simulink library "inp"  (R2021b)
settings: Solver=VariableStepAuto  StartTime=0.0  StopTime=10.0  RelTol=1e-3
undefined symbols (not defined in the file): C_TASK_5MS_S, FALSE, KINP_AcoreReadyToSlp_flg_ovrdflg, KINP_AcoreReadyToSlp_flg_ovrdval, KINP_AllowMovThd_OTA_enum_ovrdflg, KINP_AllowMovThd_OTA_enum_ovrdval, KINP_APSAngleTarget_Deg_ovrdflg, KINP_APSAngleTarget_Deg_ovrdval, KINP_APSDecReq_mps2_ovrdflg, KINP_APSDecReq_mps2_ovrdval, KINP_APSDecReqA_flg_ovrdflg, KINP_APSDecReqA_flg_ovrdval, KINP_APSDFLL_cm_ovrdflg, KINP_APSDFLL_cm_ovrdval, KINP_APSDFLR_cm_ovrdflg, KINP_APSDFLR_cm_ovrdval, KINP_APSDRLL_cm_ovrdflg, KINP_APSDRLL_cm_ovrdval, KINP_APSDRLR_cm_ovrdflg, KINP_APSDRLR_cm_ovrdval, KINP_APSExitCondition_enum_ovrdflg, KINP_APSExitCondition_enum_ovrdval, KINP_APSHWVer_enum_ovrdflg, KINP_APSHWVer_enum_ovrdval, KINP_APSProgressPCT_pct_ovrdflg, KINP_APSProgressPCT_pct_ovrdval, KINP_APSPwrReq_enum_ovrdflg, KINP_APSPwrReq_enum_ovrdval, KINP_APSReq_enum_ovrdflg, KINP_APSReq_enum_ovrdval, KINP_APSRQDisplay_enum_ovrdflg, KINP_APSRQDisplay_enum_ovrdval, KINP_APSRqEPASCtrl_flg_ovrdflg, KINP_APSRqEPASCtrl_flg_ovrdval, KINP_APSShiftPosnReq_enum_ovrdval, KINP_APSShiftPosnReq_enum_ovrflg, KINP_APSSpeedCMD_kph_ovrdval, KINP_APSSpeedCMD_kph_ovrflg, KINP_APSStaSystem_enum_ovrdflg, KINP_APSStaSystem_enum_ovrdval, KINP_APSSWVer_enum_ovrdflg, KINP_APSSWVer_enum_ovrdval, KINP_APSVMCReqA_flg_ovrdval, KINP_APSVMCReqA_flg_ovrflg, KINP_APSVRqEPASCtrl_flg_ovrdflg, KINP_APSVRqEPASCtrl_flg_ovrdval, KINP_AuxBattVolmV_mV_ovrdflg, KINP_AuxBattVolmV_mV_ovrdval, KINP_CAASSta_enum_ovrdflg, KINP_CAASSta_enum_ovrdval, KINP_CAASVMCReqA_flg_ovrdval, KINP_CAASVMCReqA_flg_ovrflg, KINP_CAN1BusOff_flg_ovrdflg, KINP_CAN1BusOff_flg_ovrdval, KINP_CAN2BusOff_flg_ovrdflg, KINP_CAN2BusOff_flg_ovrdval, KINP_CAN3BusOff_flg_ovrdflg, KINP_CAN3BusOff_flg_ovrdval, KINP_CAN4BusOff_flg_ovrdflg, KINP_CAN4BusOff_flg_ovrdval ... (+152)
libraries: FVT_lib x1037, hcu_lib x1
(part 25 of 34)

== system inp/INP/CAN3/SignalCheck/Shifter2 ==
  BHAL_outputs : Inport
  inp_CanValid_bus : Inport  Port=2
  CSW2DimSwSta : FVT_lib/inp/can_signal_template  SystemSampleTime=-1  VariantActivationTime=update diagram  Latency=0  AutoFrameSizeCalculation=off
      link override defval: Value=KINP_CSW2DimSwSta_flg_defval
      link override ovrdflg: Value=KINP_CSW2DimSwSta_flg_ovrdflg
      link override ovrdval: Value=KINP_CSW2DimSwSta_flg_ovrdval
  CSW2FWasSwSta : FVT_lib/inp/can_signal_template  SystemSampleTime=-1  VariantActivationTime=update diagram  Latency=0  AutoFrameSizeCalculation=off
      link override defval: Value=KINP_CSW2FWasSwSta_enum_defval
      link override ovrdflg: Value=KINP_CSW2FWasSwSta_enum_ovrdflg
      link override ovrdval: Value=KINP_CSW2FWasSwSta_enum_ovrdval
  CSW2FWipSwSta : FVT_lib/inp/can_signal_template  SystemSampleTime=-1  VariantActivationTime=update diagram  Latency=0  AutoFrameSizeCalculation=off
      link override defval: Value=KINP_CSW2FWipSwSta_enum_defval
      link override ovrdflg: Value=KINP_CSW2FWipSwSta_enum_ovrdflg
      link override ovrdval: Value=KINP_CSW2FWipSwSta_enum_ovrdval
  CSW2PassSWSta : FVT_lib/inp/can_signal_template  SystemSampleTime=-1  VariantActivationTime=update diagram  Latency=0  AutoFrameSizeCalculation=off
      link override defval: Value=KINP_CSW2PassSWSta_flg_defval
      link override ovrdflg: Value=KINP_CSW2PassSWSta_flg_ovrdflg
      link override ovrdval: Value=KINP_CSW2PassSWSta_flg_ovrdval
  CSW2RWipWasSwSta : FVT_lib/inp/can_signal_template  SystemSampleTime=-1  VariantActivationTime=update diagram  Latency=0  AutoFrameSizeCalculation=off
      link override defval: Value=KINP_CSW2RWipWasSwSta_enum_defval
      link override ovrdflg: Value=KINP_CSW2RWipWasSwSta_enum_ovrdflg
      link override ovrdval: Value=KINP_CSW2RWipWasSwSta_enum_ovrdval
  CSW2TurnSwSta : FVT_lib/inp/can_signal_template  SystemSampleTime=-1  VariantActivationTime=update diagram  Latency=0  AutoFrameSizeCalculation=off
      link override defval: Value=KINP_CSW2TurnSwSta_enum_defval
      link override ovrdflg: Value=KINP_CSW2TurnSwSta_enum_ovrdflg
      link override ovrdval: Value=KINP_CSW2TurnSwSta_enum_ovrdval
  Shifter2CSErr : FVT_lib/inp/can_signal_template  SystemSampleTime=-1  VariantActivationTime=update diagram  Latency=0  AutoFrameSizeCalculation=off
      link override defval: Value=KINP_Shifter2CSErr_flg_defval
      link override ovrdflg: Value=KINP_Shifter2CSErr_flg_ovrdflg
      link override ovrdval: Value=KINP_Shifter2CSErr_flg_ovrdval
  Shifter2RCErr : FVT_lib/inp/can_signal_template  SystemSampleTime=-1  VariantActivationTime=update diagram  Latency=0  AutoFrameSizeCalculation=off
      link override defval: Value=KINP_Shifter2RCErr_flg_defval
      link override ovrdflg: Value=KINP_Shifter2RCErr_flg_ovrdflg
      link override ovrdval: Value=KINP_Shifter2RCErr_flg_ovrdval
  Terminator_{1..8} (8 alike) : Terminator
  True_VHAL_CSW2DimSwSta_flg : Constant  Value=TRUE  OutDataTypeStr=boolean
  True_VHAL_CSW2FWasSwSta_enum : Constant  Value=TRUE  OutDataTypeStr=boolean
  True_VHAL_CSW2FWipSwSta_enum : Constant  Value=TRUE  OutDataTypeStr=boolean
  True_VHAL_CSW2PassSWSta_flg : Constant  Value=TRUE  OutDataTypeStr=boolean
  True_VHAL_CSW2RWipWasSwSta_enum : Constant  Value=TRUE  OutDataTypeStr=boolean
  True_VHAL_CSW2TurnSwSta_enum : Constant  Value=TRUE  OutDataTypeStr=boolean
  True_VHAL_Shifter2CSErr_flg : Constant  Value=TRUE  OutDataTypeStr=boolean
  True_VHAL_Shifter2RCErr_flg : Constant  Value=TRUE  OutDataTypeStr=boolean
  slr1_{1..8} (8 alike) : BusSelector  OutputSignals=VINP_CANMsgValidShifter2_flg
  slr_VHAL_CSW2DimSwSta_flg : BusSelector  OutputSignals=VHAL_CSW2DimSwSta_flg
  slr_VHAL_CSW2FWasSwSta_enum : BusSelector  OutputSignals=VHAL_CSW2FWasSwSta_enum
  slr_VHAL_CSW2FWipSwSta_enum : BusSelector  OutputSignals=VHAL_CSW2FWipSwSta_enum
  slr_VHAL_CSW2PassSWSta_flg : BusSelector  OutputSignals=VHAL_CSW2PassSWSta_flg
  slr_VHAL_CSW2RWipWasSwSta_enum : BusSelector  OutputSignals=VHAL_CSW2RWipWasSwSta_enum
  slr_VHAL_CSW2TurnSwSta_enum : BusSelector  OutputSignals=VHAL_CSW2TurnSwSta_enum
  slr_VHAL_Shifter2CSErr_flg : BusSelector  OutputSignals=VHAL_Shifter2CSErr_flg
  slr_VHAL_Shifter2RCErr_flg : BusSelector  OutputSignals=VHAL_Shifter2RCErr_flg
  VINP_Shifter2CSErr_flg : Outport
  VINP_Shifter2RCErr_flg : Outport  Port=2
  VINP_CSW2DimSwSta_flg : Outport  Port=3
  VINP_CSW2FWasSwSta_enum : Outport  Port=4
  VINP_CSW2FWipSwSta_enum : Outport  Port=5
  VINP_CSW2PassSWSta_flg : Outport  Port=6
  VINP_CSW2RWipWasSwSta_enum : Outport  Port=7
  VINP_CSW2TurnSwSta_enum : Outport  Port=8
  wires:
  BHAL_outputs/1 -> [BHAL_outputs]
  inp_CanValid_bus/1 -> [inp_CanValid_bus]
  [BHAL_outputs] -> slr_VHAL_Shifter2CSErr_flg/1
  slr_VHAL_Shifter2CSErr_flg/1 -> Shifter2CSErr/1  "<VHAL_Shifter2CSErr_flg>"
  True_VHAL_Shifter2CSErr_flg/1 -> Shifter2CSErr/2
  [inp_CanValid_bus] -> slr1_1/1
  slr1_1/1 -> Shifter2CSErr/3  "<VINP_CANMsgValidShifter2_flg>"
  Shifter2CSErr/1 -> VINP_Shifter2CSErr_flg/1  "VINP_Shifter2CSErr_flg"
  Shifter2CSErr/2 -> Terminator_1/1
  [BHAL_outputs] -> slr_VHAL_Shifter2RCErr_flg/1
  slr_VHAL_Shifter2RCErr_flg/1 -> Shifter2RCErr/1  "<VHAL_Shifter2RCErr_flg>"
  True_VHAL_Shifter2RCErr_flg/1 -> Shifter2RCErr/2
  [inp_CanValid_bus] -> slr1_2/1
  slr1_2/1 -> Shifter2RCErr/3  "<VINP_CANMsgValidShifter2_flg>"
  Shifter2RCErr/1 -> VINP_Shifter2RCErr_flg/1  "VINP_Shifter2RCErr_flg"
  Shifter2RCErr/2 -> Terminator_2/1
  [BHAL_outputs] -> slr_VHAL_CSW2DimSwSta_flg/1
  slr_VHAL_CSW2DimSwSta_flg/1 -> CSW2DimSwSta/1  "<VHAL_CSW2DimSwSta_flg>"
  True_VHAL_CSW2DimSwSta_flg/1 -> CSW2DimSwSta/2
  [inp_CanValid_bus] -> slr1_3/1
  slr1_3/1 -> CSW2DimSwSta/3  "<VINP_CANMsgValidShifter2_flg>"
  CSW2DimSwSta/1 -> VINP_CSW2DimSwSta_flg/1  "VINP_CSW2DimSwSta_flg"
  CSW2DimSwSta/2 -> Terminator_3/1
  [BHAL_outputs] -> slr_VHAL_CSW2FWasSwSta_enum/1
  slr_VHAL_CSW2FWasSwSta_enum/1 -> CSW2FWasSwSta/1  "<VHAL_CSW2FWasSwSta_enum>"
  True_VHAL_CSW2FWasSwSta_enum/1 -> CSW2FWasSwSta/2
  [inp_CanValid_bus] -> slr1_4/1
  slr1_4/1 -> CSW2FWasSwSta/3  "<VINP_CANMsgValidShifter2_flg>"
  CSW2FWasSwSta/1 -> VINP_CSW2FWasSwSta_enum/1  "VINP_CSW2FWasSwSta_enum"
  CSW2FWasSwSta/2 -> Terminator_4/1
  [BHAL_outputs] -> slr_VHAL_CSW2FWipSwSta_enum/1
  slr_VHAL_CSW2FWipSwSta_enum/1 -> CSW2FWipSwSta/1  "<VHAL_CSW2FWipSwSta_enum>"
  True_VHAL_CSW2FWipSwSta_enum/1 -> CSW2FWipSwSta/2
  [inp_CanValid_bus] -> slr1_5/1
  slr1_5/1 -> CSW2FWipSwSta/3  "<VINP_CANMsgValidShifter2_flg>"
  CSW2FWipSwSta/1 -> VINP_CSW2FWipSwSta_enum/1  "VINP_CSW2FWipSwSta_enum"
  CSW2FWipSwSta/2 -> Terminator_5/1
  [BHAL_outputs] -> slr_VHAL_CSW2PassSWSta_flg/1
  slr_VHAL_CSW2PassSWSta_flg/1 -> CSW2PassSWSta/1  "<VHAL_CSW2PassSWSta_flg>"
  True_VHAL_CSW2PassSWSta_flg/1 -> CSW2PassSWSta/2
  [inp_CanValid_bus] -> slr1_6/1
  slr1_6/1 -> CSW2PassSWSta/3  "<VINP_CANMsgValidShifter2_flg>"
  CSW2PassSWSta/1 -> VINP_CSW2PassSWSta_flg/1  "VINP_CSW2PassSWSta_flg"
  CSW2PassSWSta/2 -> Terminator_6/1
  [BHAL_outputs] -> slr_VHAL_CSW2RWipWasSwSta_enum/1
  slr_VHAL_CSW2RWipWasSwSta_enum/1 -> CSW2RWipWasSwSta/1  "<VHAL_CSW2RWipWasSwSta_enum>"
  True_VHAL_CSW2RWipWasSwSta_enum/1 -> CSW2RWipWasSwSta/2
  [inp_CanValid_bus] -> slr1_7/1
  slr1_7/1 -> CSW2RWipWasSwSta/3  "<VINP_CANMsgValidShifter2_flg>"
  CSW2RWipWasSwSta/1 -> VINP_CSW2RWipWasSwSta_enum/1  "VINP_CSW2RWipWasSwSta_enum"
  CSW2RWipWasSwSta/2 -> Terminator_7/1
  [BHAL_outputs] -> slr_VHAL_CSW2TurnSwSta_enum/1
  slr_VHAL_CSW2TurnSwSta_enum/1 -> CSW2TurnSwSta/1  "<VHAL_CSW2TurnSwSta_enum>"
  True_VHAL_CSW2TurnSwSta_enum/1 -> CSW2TurnSwSta/2
  [inp_CanValid_bus] -> slr1_8/1
  slr1_8/1 -> CSW2TurnSwSta/3  "<VINP_CANMsgValidShifter2_flg>"
  CSW2TurnSwSta/1 -> VINP_CSW2TurnSwSta_enum/1  "VINP_CSW2TurnSwSta_enum"
  CSW2TurnSwSta/2 -> Terminator_8/1

== system inp/INP/CAN4/SignalCheck/BodyZone_DR1 ==
  BHAL_outputs : Inport
  inp_CanValid_bus : Inport  Port=2
  BDDSEATAntiSta : FVT_lib/inp/can_signal_template  SystemSampleTime=-1  VariantActivationTime=update diagram  Latency=0  AutoFrameSizeCalculation=off
      link override defval: Value=KINP_BDDSEATAntiSta_flg_defval
      link override ovrdflg: Value=KINP_BDDSEATAntiSta_flg_ovrdflg
      link override ovrdval: Value=KINP_BDDSEATAntiSta_flg_ovrdval
  BDDSEATEntryFunSta : FVT_lib/inp/can_signal_template  SystemSampleTime=-1  VariantActivationTime=update diagram  Latency=0  AutoFrameSizeCalculation=off
      link override defval: Value=KINP_BDDSEATEntryFunSta_flg_defval
      link override ovrdflg: Value=KINP_BDDSEATEntryFunSta_flg_ovrdflg
      link override ovrdval: Value=KINP_BDDSEATEntryFunSta_flg_ovrdval
  BDDSEATErrorSta : FVT_lib/inp/can_signal_template  SystemSampleTime=-1  VariantActivationTime=update diagram  Latency=0  AutoFrameSizeCalculation=off
      link override defval: Value=KINP_BDDSEATErrorSta_flg_defval
      link override ovrdflg: Value=KINP_BDDSEATErrorSta_flg_ovrdflg
      link override ovrdval: Value=KINP_BDDSEATErrorSta_flg_ovrdval
  BDDSEATMemSetSta : FVT_lib/inp/can_signal_template  SystemSampleTime=-1  VariantActivationTime=update diagram  Latency=0  AutoFrameSizeCalculation=off
      link override defval: Value=KINP_BDDSEATMemSetSta_enum_defval
      link override ovrdflg: Value=KINP_BDDSEATMemSetSta_enum_ovrdflg
      link override ovrdval: Value=KINP_BDDSEATMemSetSta_enum_ovrdval
  BDDSEATModeSta : FVT_lib/inp/can_signal_template  SystemSampleTime=-1  VariantActivationTime=update diagram  Latency=0  AutoFrameSizeCalculation=off
      link override defval: Value=KINP_BDDSEATModeSta_enum_defval
      link override ovrdflg: Value=KINP_BDDSEATModeSta_enum_ovrdflg
      link override ovrdval: Value=KINP_BDDSEATModeSta_enum_ovrdval
  BDDSEATVentSta : FVT_lib/inp/can_signal_template  SystemSampleTime=-1  VariantActivationTime=update diagram  Latency=0  AutoFrameSizeCalculation=off
      link override defval: Value=KINP_BDDSEATVentSta_enum_defval
      link override ovrdflg: Value=KINP_BDDSEATVentSta_enum_ovrdflg
      link override ovrdval: Value=KINP_BDDSEATVentSta_enum_ovrdval
  BDDSEATheaterSta : FVT_lib/inp/can_signal_template  SystemSampleTime=-1  VariantActivationTime=update diagram  Latency=0  AutoFrameSizeCalculation=off
      link override defval: Value=KINP_BDDSEATheaterSta_enum_defval
      link override ovrdflg: Value=KINP_BDDSEATheaterSta_enum_ovrdflg
      link override ovrdval: Value=KINP_BDDSEATheaterSta_enum_ovrdval
  Terminator_{1..7} (7 alike) : Terminator
  True_VHAL_BDDSEATAntiSta_flg : Constant  Value=TRUE  OutDataTypeStr=boolean
  True_VHAL_BDDSEATEntryFunSta_flg : Constant  Value=TRUE  OutDataTypeStr=boolean
  True_VHAL_BDDSEATErrorSta_flg : Constant  Value=TRUE  OutDataTypeStr=boolean
  True_VHAL_BDDSEATMemSetSta_enum : Constant  Value=TRUE  OutDataTypeStr=boolean
  True_VHAL_BDDSEATModeSta_enum : Constant  Value=TRUE  OutDataTypeStr=boolean
  True_VHAL_BDDSEATVentSta_enum : Constant  Value=TRUE  OutDataTypeStr=boolean
  True_VHAL_BDDSEATheaterSta_enum : Constant  Value=TRUE  OutDataTypeStr=boolean
  slr1_{1..7} (7 alike) : BusSelector  OutputSignals=VINP_CANMsgValidBodyZoneDR1_flg
  slr_VHAL_BDDSEATAntiSta_flg : BusSelector  OutputSignals=VHAL_BDDSEATAntiSta_flg
  slr_VHAL_BDDSEATEntryFunSta_flg : BusSelector  OutputSignals=VHAL_BDDSEATEntryFunSta_flg
  slr_VHAL_BDDSEATErrorSta_flg : BusSelector  OutputSignals=VHAL_BDDSEATErrorSta_flg
  slr_VHAL_BDDSEATMemSetSta_enum : BusSelector  OutputSignals=VHAL_BDDSEATMemSetSta_enum
  slr_VHAL_BDDSEATModeSta_enum : BusSelector  OutputSignals=VHAL_BDDSEATModeSta_enum
  slr_VHAL_BDDSEATVentSta_enum : BusSelector  OutputSignals=VHAL_BDDSEATVentSta_enum
  slr_VHAL_BDDSEATheaterSta_enum : BusSelector  OutputSignals=VHAL_BDDSEATheaterSta_enum
  VINP_BDDSEATAntiSta_flg : Outport
  VINP_BDDSEATEntryFunSta_flg : Outport  Port=2
  VINP_BDDSEATErrorSta_flg : Outport  Port=3
  VINP_BDDSEATMemSetSta_enum : Outport  Port=4
  VINP_BDDSEATModeSta_enum : Outport  Port=5
  VINP_BDDSEATVentSta_enum : Outport  Port=6
  VINP_BDDSEATheaterSta_enum : Outport  Port=7
  wires:
  BHAL_outputs/1 -> [BHAL_outputs]
  inp_CanValid_bus/1 -> [inp_CanValid_bus]
  [BHAL_outputs] -> slr_VHAL_BDDSEATAntiSta_flg/1
  slr_VHAL_BDDSEATAntiSta_flg/1 -> BDDSEATAntiSta/1  "<VHAL_BDDSEATAntiSta_flg>"
  True_VHAL_BDDSEATAntiSta_flg/1 -> BDDSEATAntiSta/2
  [inp_CanValid_bus] -> slr1_1/1
  slr1_1/1 -> BDDSEATAntiSta/3  "<VINP_CANMsgValidBodyZoneDR1_flg>"
  BDDSEATAntiSta/1 -> VINP_BDDSEATAntiSta_flg/1  "VINP_BDDSEATAntiSta_flg"
  BDDSEATAntiSta/2 -> Terminator_1/1
  [BHAL_outputs] -> slr_VHAL_BDDSEATEntryFunSta_flg/1
  slr_VHAL_BDDSEATEntryFunSta_flg/1 -> BDDSEATEntryFunSta/1  "<VHAL_BDDSEATEntryFunSta_flg>"
  True_VHAL_BDDSEATEntryFunSta_flg/1 -> BDDSEATEntryFunSta/2
  [inp_CanValid_bus] -> slr1_2/1
  slr1_2/1 -> BDDSEATEntryFunSta/3  "<VINP_CANMsgValidBodyZoneDR1_flg>"
  BDDSEATEntryFunSta/1 -> VINP_BDDSEATEntryFunSta_flg/1  "VINP_BDDSEATEntryFunSta_flg"
  BDDSEATEntryFunSta/2 -> Terminator_2/1
  [BHAL_outputs] -> slr_VHAL_BDDSEATErrorSta_flg/1
  slr_VHAL_BDDSEATErrorSta_flg/1 -> BDDSEATErrorSta/1  "<VHAL_BDDSEATErrorSta_flg>"
  True_VHAL_BDDSEATErrorSta_flg/1 -> BDDSEATErrorSta/2
  [inp_CanValid_bus] -> slr1_3/1
  slr1_3/1 -> BDDSEATErrorSta/3  "<VINP_CANMsgValidBodyZoneDR1_flg>"
  BDDSEATErrorSta/1 -> VINP_BDDSEATErrorSta_flg/1  "VINP_BDDSEATErrorSta_flg"
  BDDSEATErrorSta/2 -> Terminator_3/1
  [BHAL_outputs] -> slr_VHAL_BDDSEATMemSetSta_enum/1
  slr_VHAL_BDDSEATMemSetSta_enum/1 -> BDDSEATMemSetSta/1  "<VHAL_BDDSEATMemSetSta_enum>"
  True_VHAL_BDDSEATMemSetSta_enum/1 -> BDDSEATMemSetSta/2
  [inp_CanValid_bus] -> slr1_4/1
  slr1_4/1 -> BDDSEATMemSetSta/3  "<VINP_CANMsgValidBodyZoneDR1_flg>"
  BDDSEATMemSetSta/1 -> VINP_BDDSEATMemSetSta_enum/1  "VINP_BDDSEATMemSetSta_enum"
  BDDSEATMemSetSta/2 -> Terminator_4/1
  [BHAL_outputs] -> slr_VHAL_BDDSEATModeSta_enum/1
  slr_VHAL_BDDSEATModeSta_enum/1 -> BDDSEATModeSta/1  "<VHAL_BDDSEATModeSta_enum>"
  True_VHAL_BDDSEATModeSta_enum/1 -> BDDSEATModeSta/2
  [inp_CanValid_bus] -> slr1_5/1
  slr1_5/1 -> BDDSEATModeSta/3  "<VINP_CANMsgValidBodyZoneDR1_flg>"
  BDDSEATModeSta/1 -> VINP_BDDSEATModeSta_enum/1  "VINP_BDDSEATModeSta_enum"
  BDDSEATModeSta/2 -> Terminator_5/1
  [BHAL_outputs] -> slr_VHAL_BDDSEATVentSta_enum/1
  slr_VHAL_BDDSEATVentSta_enum/1 -> BDDSEATVentSta/1  "<VHAL_BDDSEATVentSta_enum>"
  True_VHAL_BDDSEATVentSta_enum/1 -> BDDSEATVentSta/2
  [inp_CanValid_bus] -> slr1_6/1
  slr1_6/1 -> BDDSEATVentSta/3  "<VINP_CANMsgValidBodyZoneDR1_flg>"
  BDDSEATVentSta/1 -> VINP_BDDSEATVentSta_enum/1  "VINP_BDDSEATVentSta_enum"
  BDDSEATVentSta/2 -> Terminator_6/1
  [BHAL_outputs] -> slr_VHAL_BDDSEATheaterSta_enum/1
  slr_VHAL_BDDSEATheaterSta_enum/1 -> BDDSEATheaterSta/1  "<VHAL_BDDSEATheaterSta_enum>"
  True_VHAL_BDDSEATheaterSta_enum/1 -> BDDSEATheaterSta/2
  [inp_CanValid_bus] -> slr1_7/1
  slr1_7/1 -> BDDSEATheaterSta/3  "<VINP_CANMsgValidBodyZoneDR1_flg>"
  BDDSEATheaterSta/1 -> VINP_BDDSEATheaterSta_enum/1  "VINP_BDDSEATheaterSta_enum"
  BDDSEATheaterSta/2 -> Terminator_7/1

== system inp/INP/CAN4/SignalCheck/BodyZone_DR2 ==
  BHAL_outputs : Inport
  inp_CanValid_bus : Inport  Port=2
  BDAPMWinFOpenedSta : FVT_lib/inp/can_signal_template  SystemSampleTime=-1  VariantActivationTime=update diagram  Latency=0  AutoFrameSizeCalculation=off
      link override defval: Value=KINP_BDAPMWinFOpenedSta_pct_defval
      link override ovrdflg: Value=KINP_BDAPMWinFOpenedSta_pct_ovrdflg
      link override ovrdval: Value=KINP_BDAPMWinFOpenedSta_pct_ovrdval
  BDAPMWinROpenedSta : FVT_lib/inp/can_signal_template  SystemSampleTime=-1  VariantActivationTime=update diagram  Latency=0  AutoFrameSizeCalculation=off
      link override defval: Value=KINP_BDAPMWinROpenedSta_pct_defval
      link override ovrdflg: Value=KINP_BDAPMWinROpenedSta_pct_ovrdflg
      link override ovrdval: Value=KINP_BDAPMWinROpenedSta_pct_ovrdval
  BDDoorFHandleCloseSta : FVT_lib/inp/can_signal_template  SystemSampleTime=-1  VariantActivationTime=update diagram  Latency=0  AutoFrameSizeCalculation=off
      link override defval: Value=KINP_BDDoorFHandleCloseSta_flg_defval
      link override ovrdflg: Value=KINP_BDDoorFHandleCloseSta_flg_ovrdflg
      link override ovrdval: Value=KINP_BDDoorFHandleCloseSta_flg_ovrdval
  BDDoorRHandleCloseSta : FVT_lib/inp/can_signal_template  SystemSampleTime=-1  VariantActivationTime=update diagram  Latency=0  AutoFrameSizeCalculation=off
      link override defval: Value=KINP_BDDoorRHandleCloseSta_flg_defval
      link override ovrdflg: Value=KINP_BDDoorRHandleCloseSta_flg_ovrdflg
      link override ovrdval: Value=KINP_BDDoorRHandleCloseSta_flg_ovrdval
  Terminator_{1..4} (4 alike) : Terminator
  True_VHAL_BDAPMWinFOpenedSta_pct : Constant  Value=TRUE  OutDataTypeStr=boolean
  True_VHAL_BDAPMWinROpenedSta_pct : Constant  Value=TRUE  OutDataTypeStr=boolean
  True_VHAL_BDDoorFHandleCloseSta_flg : Constant  Value=TRUE  OutDataTypeStr=boolean
  True_VHAL_BDDoorRHandleCloseSta_flg : Constant  Value=TRUE  OutDataTypeStr=boolean
  slr1_{1..4} (4 alike) : BusSelector  OutputSignals=VINP_CANMsgValidBodyZoneDR2_flg
  slr_VHAL_BDAPMWinFOpenedSta_pct : BusSelector  OutputSignals=VHAL_BDAPMWinFOpenedSta_pct
  slr_VHAL_BDAPMWinROpenedSta_pct : BusSelector  OutputSignals=VHAL_BDAPMWinROpenedSta_pct
  slr_VHAL_BDDoorFHandleCloseSta_flg : BusSelector  OutputSignals=VHAL_BDDoorFHandleCloseSta_flg
  slr_VHAL_BDDoorRHandleCloseSta_flg : BusSelector  OutputSignals=VHAL_BDDoorRHandleCloseSta_flg
  VINP_BDAPMWinFOpenedSta_pct : Outport
  VINP_BDAPMWinROpenedSta_pct : Outport  Port=2
  VINP_BDDoorFHandleCloseSta_flg : Outport  Port=3
  VINP_BDDoorRHandleCloseSta_flg : Outport  Port=4
  wires:
  BHAL_outputs/1 -> [BHAL_outputs]
  inp_CanValid_bus/1 -> [inp_CanValid_bus]
  [BHAL_outputs] -> slr_VHAL_BDAPMWinFOpenedSta_pct/1
  slr_VHAL_BDAPMWinFOpenedSta_pct/1 -> BDAPMWinFOpenedSta/1  "<VHAL_BDAPMWinFOpenedSta_pct>"
  True_VHAL_BDAPMWinFOpenedSta_pct/1 -> BDAPMWinFOpenedSta/2
  [inp_CanValid_bus] -> slr1_1/1
  slr1_1/1 -> BDAPMWinFOpenedSta/3  "<VINP_CANMsgValidBodyZoneDR2_flg>"
  BDAPMWinFOpenedSta/1 -> VINP_BDAPMWinFOpenedSta_pct/1  "VINP_BDAPMWinFOpenedSta_pct"
  BDAPMWinFOpenedSta/2 -> Terminator_1/1
  [BHAL_outputs] -> slr_VHAL_BDAPMWinROpenedSta_pct/1
  slr_VHAL_BDAPMWinROpenedSta_pct/1 -> BDAPMWinROpenedSta/1  "<VHAL_BDAPMWinROpenedSta_pct>"
  True_VHAL_BDAPMWinROpenedSta_pct/1 -> BDAPMWinROpenedSta/2
  [inp_CanValid_bus] -> slr1_2/1
  slr1_2/1 -> BDAPMWinROpenedSta/3  "<VINP_CANMsgValidBodyZoneDR2_flg>"
  BDAPMWinROpenedSta/1 -> VINP_BDAPMWinROpenedSta_pct/1  "VINP_BDAPMWinROpenedSta_pct"
  BDAPMWinROpenedSta/2 -> Terminator_2/1
  [BHAL_outputs] -> slr_VHAL_BDDoorFHandleCloseSta_flg/1
  slr_VHAL_BDDoorFHandleCloseSta_flg/1 -> BDDoorFHandleCloseSta/1  "<VHAL_BDDoorFHandleCloseSta_flg>"
  True_VHAL_BDDoorFHandleCloseSta_flg/1 -> BDDoorFHandleCloseSta/2
  [inp_CanValid_bus] -> slr1_3/1
  slr1_3/1 -> BDDoorFHandleCloseSta/3  "<VINP_CANMsgValidBodyZoneDR2_flg>"
  BDDoorFHandleCloseSta/1 -> VINP_BDDoorFHandleCloseSta_flg/1  "VINP_BDDoorFHandleCloseSta_flg"
  BDDoorFHandleCloseSta/2 -> Terminator_3/1
  [BHAL_outputs] -> slr_VHAL_BDDoorRHandleCloseSta_flg/1
  slr_VHAL_BDDoorRHandleCloseSta_flg/1 -> BDDoorRHandleCloseSta/1  "<VHAL_BDDoorRHandleCloseSta_flg>"
  True_VHAL_BDDoorRHandleCloseSta_flg/1 -> BDDoorRHandleCloseSta/2
  [inp_CanValid_bus] -> slr1_4/1
  slr1_4/1 -> BDDoorRHandleCloseSta/3  "<VINP_CANMsgValidBodyZoneDR2_flg>"
  BDDoorRHandleCloseSta/1 -> VINP_BDDoorRHandleCloseSta_flg/1  "VINP_BDDoorRHandleCloseSta_flg"
  BDDoorRHandleCloseSta/2 -> Terminator_4/1

== system inp/INP/CAN4/SignalCheck/BodyZone_PS1 ==
  BHAL_outputs : Inport
  inp_CanValid_bus : Inport  Port=2
  BPPSEATErrorSta : FVT_lib/inp/can_signal_template  SystemSampleTime=-1  VariantActivationTime=update diagram  Latency=0  AutoFrameSizeCalculation=off
      link override defval: Value=KINP_BPPSEATErrorSta_flg_defval
      link override ovrdflg: Value=KINP_BPPSEATErrorSta_flg_ovrdflg
      link override ovrdval: Value=KINP_BPPSEATErrorSta_flg_ovrdval
  BPPSEATModeSta : FVT_lib/inp/can_signal_template  SystemSampleTime=-1  VariantActivationTime=update diagram  Latency=0  AutoFrameSizeCalculation=off
      link override defval: Value=KINP_BPPSEATModeSta_enum_defval
      link override ovrdflg: Value=KINP_BPPSEATModeSta_enum_ovrdflg
      link override ovrdval: Value=KINP_BPPSEATModeSta_enum_ovrdval
  BPPSEATVentSta : FVT_lib/inp/can_signal_template  SystemSampleTime=-1  VariantActivationTime=update diagram  Latency=0  AutoFrameSizeCalculation=off
      link override defval: Value=KINP_BPPSEATVentSta_enum_defval
      link override ovrdflg: Value=KINP_BPPSEATVentSta_enum_ovrdflg
      link override ovrdval: Value=KINP_BPPSEATVentSta_enum_ovrdval
  BPPSEATheaterSta : FVT_lib/inp/can_signal_template  SystemSampleTime=-1  VariantActivationTime=update diagram  Latency=0  AutoFrameSizeCalculation=off
      link override defval: Value=KINP_BPPSEATheaterSta_enum_defval
      link override ovrdflg: Value=KINP_BPPSEATheaterSta_enum_ovrdflg
      link override ovrdval: Value=KINP_BPPSEATheaterSta_enum_ovrdval
  BPPTGActiveSta : FVT_lib/inp/can_signal_template  SystemSampleTime=-1  VariantActivationTime=update diagram  Latency=0  AutoFrameSizeCalculation=off
      link override defval: Value=KINP_BPPTGActiveSta_enum_defval
      link override ovrdflg: Value=KINP_BPPTGActiveSta_enum_ovrdflg
      link override ovrdval: Value=KINP_BPPTGActiveSta_enum_ovrdval
  BPPTGExistSta : FVT_lib/inp/can_signal_template  SystemSampleTime=-1  VariantActivationTime=update diagram  Latency=0  AutoFrameSizeCalculation=off
      link override defval: Value=KINP_BPPTGExistSta_flg_defval
      link override ovrdflg: Value=KINP_BPPTGExistSta_flg_ovrdflg
      link override ovrdval: Value=KINP_BPPTGExistSta_flg_ovrdval
  BPPTGInsideSW1Sta : FVT_lib/inp/can_signal_template  SystemSampleTime=-1  VariantActivationTime=update diagram  Latency=0  AutoFrameSizeCalculation=off
      link override defval: Value=KINP_BPPTGInsideSW1Sta_enum_defval
      link override ovrdflg: Value=KINP_BPPTGInsideSW1Sta_enum_ovrdflg
      link override ovrdval: Value=KINP_BPPTGInsideSW1Sta_enum_ovrdval
  BPPTGInsideSW2Sta : FVT_lib/inp/can_signal_template  SystemSampleTime=-1  VariantActivationTime=update diagram  Latency=0  AutoFrameSizeCalculation=off
      link override defval: Value=KINP_BPPTGInsideSW2Sta_enum_defval
      link override ovrdflg: Value=KINP_BPPTGInsideSW2Sta_enum_ovrdflg
      link override ovrdval: Value=KINP_BPPTGInsideSW2Sta_enum_ovrdval
  BPPTGIsSetHeightSta : FVT_lib/inp/can_signal_template  SystemSampleTime=-1  VariantActivationTime=update diagram  Latency=0  AutoFrameSizeCalculation=off
      link override defval: Value=KINP_BPPTGIsSetHeightSta_flg_defval
      link override ovrdflg: Value=KINP_BPPTGIsSetHeightSta_flg_ovrdflg
      link override ovrdval: Value=KINP_BPPTGIsSetHeightSta_flg_ovrdval
  BPPTGLeftHallPosnSta : FVT_lib/inp/can_signal_template  SystemSampleTime=-1  VariantActivationTime=update diagram  Latency=0  AutoFrameSizeCalculation=off
      link override defval: Value=KINP_BPPTGLeftHallPosnSta_enum_defval
      link override ovrdflg: Value=KINP_BPPTGLeftHallPosnSta_enum_ovrdflg
      link override ovrdval: Value=KINP_BPPTGLeftHallPosnSta_enum_ovrdval
  BPPTGOpenRatioSta : FVT_lib/inp/can_signal_template  SystemSampleTime=-1  VariantActivationTime=update diagram  Latency=0  AutoFrameSizeCalculation=off
      link override defval: Value=KINP_BPPTGOpenRatioSta_pct_defval
      link override ovrdflg: Value=KINP_BPPTGOpenRatioSta_pct_ovrdflg
      link override ovrdval: Value=KINP_BPPTGOpenRatioSta_pct_ovrdval
  BPPTGRDILCmd : FVT_lib/inp/can_signal_template  SystemSampleTime=-1  VariantActivationTime=update diagram  Latency=0  AutoFrameSizeCalculation=off
      link override defval: Value=KINP_BPPTGRDILCmd_enum_defval
      link override ovrdflg: Value=KINP_BPPTGRDILCmd_enum_ovrdflg
      link override ovrdval: Value=KINP_BPPTGRDILCmd_enum_ovrdval
  BPPTGSysSta : FVT_lib/inp/can_signal_template  SystemSampleTime=-1  VariantActivationTime=update diagram  Latency=0  AutoFrameSizeCalculation=off
      link override defval: Value=KINP_BPPTGSysSta_enum_defval
      link override ovrdflg: Value=KINP_BPPTGSysSta_enum_ovrdflg
      link override ovrdval: Value=KINP_BPPTGSysSta_enum_ovrdval
  Terminator_{1..13} (13 alike) : Terminator
  True_VHAL_BPPSEATErrorSta_flg : Constant  Value=TRUE  OutDataTypeStr=boolean
  True_VHAL_BPPSEATModeSta_enum : Constant  Value=TRUE  OutDataTypeStr=boolean
  True_VHAL_BPPSEATVentSta_enum : Constant  Value=TRUE  OutDataTypeStr=boolean
  True_VHAL_BPPSEATheaterSta_enum : Constant  Value=TRUE  OutDataTypeStr=boolean
  True_VHAL_BPPTGActiveSta_enum : Constant  Value=TRUE  OutDataTypeStr=boolean
  True_VHAL_BPPTGExistSta_flg : Constant  Value=TRUE  OutDataTypeStr=boolean
  True_VHAL_BPPTGInsideSW1Sta_enum : Constant  Value=TRUE  OutDataTypeStr=boolean
  True_VHAL_BPPTGInsideSW2Sta_enum : Constant  Value=TRUE  OutDataTypeStr=boolean
  True_VHAL_BPPTGIsSetHeightSta_flg : Constant  Value=TRUE  OutDataTypeStr=boolean
  True_VHAL_BPPTGLeftHallPosnSta_enum : Constant  Value=TRUE  OutDataTypeStr=boolean
  True_VHAL_BPPTGOpenRatioSta_pct : Constant  Value=TRUE  OutDataTypeStr=boolean
  True_VHAL_BPPTGRDILCmd_enum : Constant  Value=TRUE  OutDataTypeStr=boolean
  True_VHAL_BPPTGSysSta_enum : Constant  Value=TRUE  OutDataTypeStr=boolean
  slr1_{1..13} (13 alike) : BusSelector  OutputSignals=VINP_CANMsgValidBodyZonePS1_flg
  slr_VHAL_BPPSEATErrorSta_flg : BusSelector  OutputSignals=VHAL_BPPSEATErrorSta_flg
  slr_VHAL_BPPSEATModeSta_enum : BusSelector  OutputSignals=VHAL_BPPSEATModeSta_enum
  slr_VHAL_BPPSEATVentSta_enum : BusSelector  OutputSignals=VHAL_BPPSEATVentSta_enum
  slr_VHAL_BPPSEATheaterSta_enum : BusSelector  OutputSignals=VHAL_BPPSEATheaterSta_enum
  slr_VHAL_BPPTGActiveSta_enum : BusSelector  OutputSignals=VHAL_BPPTGActiveSta_enum
  slr_VHAL_BPPTGExistSta_flg : BusSelector  OutputSignals=VHAL_BPPTGExistSta_flg
  slr_VHAL_BPPTGInsideSW1Sta_enum : BusSelector  OutputSignals=VHAL_BPPTGInsideSW1Sta_enum
  slr_VHAL_BPPTGInsideSW2Sta_enum : BusSelector  OutputSignals=VHAL_BPPTGInsideSW2Sta_enum
  slr_VHAL_BPPTGIsSetHeightSta_flg : BusSelector  OutputSignals=VHAL_BPPTGIsSetHeightSta_flg
  slr_VHAL_BPPTGLeftHallPosnSta_enum : BusSelector  OutputSignals=VHAL_BPPTGLeftHallPosnSta_enum
  slr_VHAL_BPPTGOpenRatioSta_pct : BusSelector  OutputSignals=VHAL_BPPTGOpenRatioSta_pct
  slr_VHAL_BPPTGRDILCmd_enum : BusSelector  OutputSignals=VHAL_BPPTGRDILCmd_enum
  slr_VHAL_BPPTGSysSta_enum : BusSelector  OutputSignals=VHAL_BPPTGSysSta_enum
  VINP_BPPSEATErrorSta_flg : Outport
  VINP_BPPSEATModeSta_enum : Outport  Port=2
  VINP_BPPSEATVentSta_enum : Outport  Port=3
  VINP_BPPSEATheaterSta_enum : Outport  Port=4
  VINP_BPPTGActiveSta_enum : Outport  Port=5
  VINP_BPPTGExistSta_flg : Outport  Port=6
  VINP_BPPTGInsideSW1Sta_enum : Outport  Port=7
  VINP_BPPTGInsideSW2Sta_enum : Outport  Port=8
  VINP_BPPTGIsSetHeightSta_flg : Outport  Port=9
  VINP_BPPTGLeftHallPosnSta_enum : Outport  Port=10
  VINP_BPPTGOpenRatioSta_pct : Outport  Port=11
  VINP_BPPTGRDILCmd_enum : Outport  Port=12
  VINP_BPPTGSysSta_enum : Outport  Port=13
  wires:
  BHAL_outputs/1 -> [BHAL_outputs]
  inp_CanValid_bus/1 -> [inp_CanValid_bus]
  [BHAL_outputs] -> slr_VHAL_BPPSEATErrorSta_flg/1
  slr_VHAL_BPPSEATErrorSta_flg/1 -> BPPSEATErrorSta/1  "<VHAL_BPPSEATErrorSta_flg>"
  True_VHAL_BPPSEATErrorSta_flg/1 -> BPPSEATErrorSta/2
  [inp_CanValid_bus] -> slr1_1/1
  slr1_1/1 -> BPPSEATErrorSta/3  "<VINP_CANMsgValidBodyZonePS1_flg>"
  BPPSEATErrorSta/1 -> VINP_BPPSEATErrorSta_flg/1  "VINP_BPPSEATErrorSta_flg"
  BPPSEATErrorSta/2 -> Terminator_1/1
  [BHAL_outputs] -> slr_VHAL_BPPSEATModeSta_enum/1
  slr_VHAL_BPPSEATModeSta_enum/1 -> BPPSEATModeSta/1  "<VHAL_BPPSEATModeSta_enum>"
  True_VHAL_BPPSEATModeSta_enum/1 -> BPPSEATModeSta/2
  [inp_CanValid_bus] -> slr1_2/1
  slr1_2/1 -> BPPSEATModeSta/3  "<VINP_CANMsgValidBodyZonePS1_flg>"
  BPPSEATModeSta/1 -> VINP_BPPSEATModeSta_enum/1  "VINP_BPPSEATModeSta_enum"
  BPPSEATModeSta/2 -> Terminator_2/1
  [BHAL_outputs] -> slr_VHAL_BPPSEATVentSta_enum/1
  slr_VHAL_BPPSEATVentSta_enum/1 -> BPPSEATVentSta/1  "<VHAL_BPPSEATVentSta_enum>"
  True_VHAL_BPPSEATVentSta_enum/1 -> BPPSEATVentSta/2
  [inp_CanValid_bus] -> slr1_3/1
  slr1_3/1 -> BPPSEATVentSta/3  "<VINP_CANMsgValidBodyZonePS1_flg>"
  BPPSEATVentSta/1 -> VINP_BPPSEATVentSta_enum/1  "VINP_BPPSEATVentSta_enum"
  BPPSEATVentSta/2 -> Terminator_3/1
  [BHAL_outputs] -> slr_VHAL_BPPSEATheaterSta_enum/1
  slr_VHAL_BPPSEATheaterSta_enum/1 -> BPPSEATheaterSta/1  "<VHAL_BPPSEATheaterSta_enum>"
  True_VHAL_BPPSEATheaterSta_enum/1 -> BPPSEATheaterSta/2
  [inp_CanValid_bus] -> slr1_4/1
  slr1_4/1 -> BPPSEATheaterSta/3  "<VINP_CANMsgValidBodyZonePS1_flg>"
  BPPSEATheaterSta/1 -> VINP_BPPSEATheaterSta_enum/1  "VINP_BPPSEATheaterSta_enum"
  BPPSEATheaterSta/2 -> Terminator_4/1
  [BHAL_outputs] -> slr_VHAL_BPPTGActiveSta_enum/1
  slr_VHAL_BPPTGActiveSta_enum/1 -> BPPTGActiveSta/1  "<VHAL_BPPTGActiveSta_enum>"
  True_VHAL_BPPTGActiveSta_enum/1 -> BPPTGActiveSta/2
  [inp_CanValid_bus] -> slr1_5/1
  slr1_5/1 -> BPPTGActiveSta/3  "<VINP_CANMsgValidBodyZonePS1_flg>"
  BPPTGActiveSta/1 -> VINP_BPPTGActiveSta_enum/1  "VINP_BPPTGActiveSta_enum"
  BPPTGActiveSta/2 -> Terminator_5/1
  [BHAL_outputs] -> slr_VHAL_BPPTGExistSta_flg/1
  slr_VHAL_BPPTGExistSta_flg/1 -> BPPTGExistSta/1  "<VHAL_BPPTGExistSta_flg>"
  True_VHAL_BPPTGExistSta_flg/1 -> BPPTGExistSta/2
  [inp_CanValid_bus] -> slr1_6/1
  slr1_6/1 -> BPPTGExistSta/3  "<VINP_CANMsgValidBodyZonePS1_flg>"
  BPPTGExistSta/1 -> VINP_BPPTGExistSta_flg/1  "VINP_BPPTGExistSta_flg"
  BPPTGExistSta/2 -> Terminator_6/1
  [BHAL_outputs] -> slr_VHAL_BPPTGInsideSW1Sta_enum/1
  slr_VHAL_BPPTGInsideSW1Sta_enum/1 -> BPPTGInsideSW1Sta/1  "<VHAL_BPPTGInsideSW1Sta_enum>"
  True_VHAL_BPPTGInsideSW1Sta_enum/1 -> BPPTGInsideSW1Sta/2
  [inp_CanValid_bus] -> slr1_7/1
  slr1_7/1 -> BPPTGInsideSW1Sta/3  "<VINP_CANMsgValidBodyZonePS1_flg>"
  BPPTGInsideSW1Sta/1 -> VINP_BPPTGInsideSW1Sta_enum/1  "VINP_BPPTGInsideSW1Sta_enum"
  BPPTGInsideSW1Sta/2 -> Terminator_7/1
  [BHAL_outputs] -> slr_VHAL_BPPTGInsideSW2Sta_enum/1
  slr_VHAL_BPPTGInsideSW2Sta_enum/1 -> BPPTGInsideSW2Sta/1  "<VHAL_BPPTGInsideSW2Sta_enum>"
  True_VHAL_BPPTGInsideSW2Sta_enum/1 -> BPPTGInsideSW2Sta/2
  [inp_CanValid_bus] -> slr1_8/1
  slr1_8/1 -> BPPTGInsideSW2Sta/3  "<VINP_CANMsgValidBodyZonePS1_flg>"
  BPPTGInsideSW2Sta/1 -> VINP_BPPTGInsideSW2Sta_enum/1  "VINP_BPPTGInsideSW2Sta_enum"
  BPPTGInsideSW2Sta/2 -> Terminator_8/1
  [BHAL_outputs] -> slr_VHAL_BPPTGIsSetHeightSta_flg/1
  slr_VHAL_BPPTGIsSetHeightSta_flg/1 -> BPPTGIsSetHeightSta/1  "<VHAL_BPPTGIsSetHeightSta_flg>"
  True_VHAL_BPPTGIsSetHeightSta_flg/1 -> BPPTGIsSetHeightSta/2
  [inp_CanValid_bus] -> slr1_9/1
  slr1_9/1 -> BPPTGIsSetHeightSta/3  "<VINP_CANMsgValidBodyZonePS1_flg>"
  BPPTGIsSetHeightSta/1 -> VINP_BPPTGIsSetHeightSta_flg/1  "VINP_BPPTGIsSetHeightSta_flg"
  BPPTGIsSetHeightSta/2 -> Terminator_9/1
  [BHAL_outputs] -> slr_VHAL_BPPTGLeftHallPosnSta_enum/1
  slr_VHAL_BPPTGLeftHallPosnSta_enum/1 -> BPPTGLeftHallPosnSta/1  "<VHAL_BPPTGLeftHallPosnSta_enum>"
  True_VHAL_BPPTGLeftHallPosnSta_enum/1 -> BPPTGLeftHallPosnSta/2
  [inp_CanValid_bus] -> slr1_10/1
  slr1_10/1 -> BPPTGLeftHallPosnSta/3  "<VINP_CANMsgValidBodyZonePS1_flg>"
  BPPTGLeftHallPosnSta/1 -> VINP_BPPTGLeftHallPosnSta_enum/1  "VINP_BPPTGLeftHallPosnSta_enum"
  BPPTGLeftHallPosnSta/2 -> Terminator_10/1
  [BHAL_outputs] -> slr_VHAL_BPPTGOpenRatioSta_pct/1
  slr_VHAL_BPPTGOpenRatioSta_pct/1 -> BPPTGOpenRatioSta/1  "<VHAL_BPPTGOpenRatioSta_pct>"
  True_VHAL_BPPTGOpenRatioSta_pct/1 -> BPPTGOpenRatioSta/2
  [inp_CanValid_bus] -> slr1_11/1
  slr1_11/1 -> BPPTGOpenRatioSta/3  "<VINP_CANMsgValidBodyZonePS1_flg>"
  BPPTGOpenRatioSta/1 -> VINP_BPPTGOpenRatioSta_pct/1  "VINP_BPPTGOpenRatioSta_pct"
  BPPTGOpenRatioSta/2 -> Terminator_11/1
  [BHAL_outputs] -> slr_VHAL_BPPTGRDILCmd_enum/1
  slr_VHAL_BPPTGRDILCmd_enum/1 -> BPPTGRDILCmd/1  "<VHAL_BPPTGRDILCmd_enum>"
  True_VHAL_BPPTGRDILCmd_enum/1 -> BPPTGRDILCmd/2
  [inp_CanValid_bus] -> slr1_12/1
  slr1_12/1 -> BPPTGRDILCmd/3  "<VINP_CANMsgValidBodyZonePS1_flg>"
  BPPTGRDILCmd/1 -> VINP_BPPTGRDILCmd_enum/1  "VINP_BPPTGRDILCmd_enum"
  BPPTGRDILCmd/2 -> Terminator_12/1
  [BHAL_outputs] -> slr_VHAL_BPPTGSysSta_enum/1
  slr_VHAL_BPPTGSysSta_enum/1 -> BPPTGSysSta/1  "<VHAL_BPPTGSysSta_enum>"
  True_VHAL_BPPTGSysSta_enum/1 -> BPPTGSysSta/2
  [inp_CanValid_bus] -> slr1_13/1
  slr1_13/1 -> BPPTGSysSta/3  "<VINP_CANMsgValidBodyZonePS1_flg>"
  BPPTGSysSta/1 -> VINP_BPPTGSysSta_enum/1  "VINP_BPPTGSysSta_enum"
  BPPTGSysSta/2 -> Terminator_13/1

== system inp/INP/CAN4/SignalCheck/BodyZone_PS2 ==
  BHAL_outputs : Inport
  inp_CanValid_bus : Inport  Port=2
  BPAPMWinFOpenedSta : FVT_lib/inp/can_signal_template  SystemSampleTime=-1  VariantActivationTime=update diagram  Latency=0  AutoFrameSizeCalculation=off
      link override defval: Value=KINP_BPAPMWinFOpenedSta_pct_defval
      link override ovrdflg: Value=KINP_BPAPMWinFOpenedSta_pct_ovrdflg
      link override ovrdval: Value=KINP_BPAPMWinFOpenedSta_pct_ovrdval
  BPAPMWinROpenedSta : FVT_lib/inp/can_signal_template  SystemSampleTime=-1  VariantActivationTime=update diagram  Latency=0  AutoFrameSizeCalculation=off
      link override defval: Value=KINP_BPAPMWinROpenedSta_pct_defval
      link override ovrdflg: Value=KINP_BPAPMWinROpenedSta_pct_ovrdflg
      link override ovrdval: Value=KINP_BPAPMWinROpenedSta_pct_ovrdval
  BPDoorFHandleCloseSta : FVT_lib/inp/can_signal_template  SystemSampleTime=-1  VariantActivationTime=update diagram  Latency=0  AutoFrameSizeCalculation=off
      link override defval: Value=KINP_BPDoorFHandleCloseSta_flg_defval
      link override ovrdflg: Value=KINP_BPDoorFHandleCloseSta_flg_ovrdflg
      link override ovrdval: Value=KINP_BPDoorFHandleCloseSta_flg_ovrdval
  BPDoorRHandleCloseSta : FVT_lib/inp/can_signal_template  SystemSampleTime=-1  VariantActivationTime=update diagram  Latency=0  AutoFrameSizeCalculation=off
      link override defval: Value=KINP_BPDoorRHandleCloseSta_flg_defval
      link override ovrdflg: Value=KINP_BPDoorRHandleCloseSta_flg_ovrdflg
      link override ovrdval: Value=KINP_BPDoorRHandleCloseSta_flg_ovrdval
  BPSEATLVentSta : FVT_lib/inp/can_signal_template  SystemSampleTime=-1  VariantActivationTime=update diagram  Latency=0  AutoFrameSizeCalculation=off
      link override defval: Value=KINP_BPSEATLVentSta_enum_defval
      link override ovrdflg: Value=KINP_BPSEATLVentSta_enum_ovrdflg
      link override ovrdval: Value=KINP_BPSEATLVentSta_enum_ovrdval
  BPSEATMLVentSta : FVT_lib/inp/can_signal_template  SystemSampleTime=-1  VariantActivationTime=update diagram  Latency=0  AutoFrameSizeCalculation=off
      link override defval: Value=KINP_BPSEATMLVentSta_enum_defval
      link override ovrdflg: Value=KINP_BPSEATMLVentSta_enum_ovrdflg
      link override ovrdval: Value=KINP_BPSEATMLVentSta_enum_ovrdval
  BPSEATMRVentSta : FVT_lib/inp/can_signal_template  SystemSampleTime=-1  VariantActivationTime=update diagram  Latency=0  AutoFrameSizeCalculation=off
      link override defval: Value=KINP_BPSEATMRVentSta_enum_defval
      link override ovrdflg: Value=KINP_BPSEATMRVentSta_enum_ovrdflg
      link override ovrdval: Value=KINP_BPSEATMRVentSta_enum_ovrdval
  BPSEATRVentSta : FVT_lib/inp/can_signal_template  SystemSampleTime=-1  VariantActivationTime=update diagram  Latency=0  AutoFrameSizeCalculation=off
      link override defval: Value=KINP_BPSEATRVentSta_enum_defval
      link override ovrdflg: Value=KINP_BPSEATRVentSta_enum_ovrdflg
      link override ovrdval: Value=KINP_BPSEATRVentSta_enum_ovrdval
  Terminator_{1..8} (8 alike) : Terminator
  True_VHAL_BPAPMWinFOpenedSta_pct : Constant  Value=TRUE  OutDataTypeStr=boolean
  True_VHAL_BPAPMWinROpenedSta_pct : Constant  Value=TRUE  OutDataTypeStr=boolean
  True_VHAL_BPDoorFHandleCloseSta_flg : Constant  Value=TRUE  OutDataTypeStr=boolean
  True_VHAL_BPDoorRHandleCloseSta_flg : Constant  Value=TRUE  OutDataTypeStr=boolean
  True_VHAL_BPSEATLVentSta_enum : Constant  Value=TRUE  OutDataTypeStr=boolean
  True_VHAL_BPSEATMLVentSta_enum : Constant  Value=TRUE  OutDataTypeStr=boolean
  True_VHAL_BPSEATMRVentSta_enum : Constant  Value=TRUE  OutDataTypeStr=boolean
  True_VHAL_BPSEATRVentSta_enum : Constant  Value=TRUE  OutDataTypeStr=boolean
  slr1_{1..8} (8 alike) : BusSelector  OutputSignals=VINP_CANMsgValidBodyZonePS2_flg
  slr_VHAL_BPAPMWinFOpenedSta_pct : BusSelector  OutputSignals=VHAL_BPAPMWinFOpenedSta_pct
  slr_VHAL_BPAPMWinROpenedSta_pct : BusSelector  OutputSignals=VHAL_BPAPMWinROpenedSta_pct
  slr_VHAL_BPDoorFHandleCloseSta_flg : BusSelector  OutputSignals=VHAL_BPDoorFHandleCloseSta_flg
  slr_VHAL_BPDoorRHandleCloseSta_flg : BusSelector  OutputSignals=VHAL_BPDoorRHandleCloseSta_flg
  slr_VHAL_BPSEATLVentSta_enum : BusSelector  OutputSignals=VHAL_BPSEATLVentSta_enum
  slr_VHAL_BPSEATMLVentSta_enum : BusSelector  OutputSignals=VHAL_BPSEATMLVentSta_enum
  slr_VHAL_BPSEATMRVentSta_enum : BusSelector  OutputSignals=VHAL_BPSEATMRVentSta_enum
  slr_VHAL_BPSEATRVentSta_enum : BusSelector  OutputSignals=VHAL_BPSEATRVentSta_enum
  VINP_BPAPMWinFOpenedSta_pct : Outport
  VINP_BPAPMWinROpenedSta_pct : Outport  Port=2
  VINP_BPDoorFHandleCloseSta_flg : Outport  Port=3
  VINP_BPDoorRHandleCloseSta_flg : Outport  Port=4
  VINP_BPSEATLVentSta_enum : Outport  Port=5
  VINP_BPSEATMLVentSta_enum : Outport  Port=6
  VINP_BPSEATMRVentSta_enum : Outport  Port=7
  VINP_BPSEATRVentSta_enum : Outport  Port=8
  wires:
  BHAL_outputs/1 -> [BHAL_outputs]
  inp_CanValid_bus/1 -> [inp_CanValid_bus]
  [BHAL_outputs] -> slr_VHAL_BPAPMWinFOpenedSta_pct/1
  slr_VHAL_BPAPMWinFOpenedSta_pct/1 -> BPAPMWinFOpenedSta/1  "<VHAL_BPAPMWinFOpenedSta_pct>"
  True_VHAL_BPAPMWinFOpenedSta_pct/1 -> BPAPMWinFOpenedSta/2
  [inp_CanValid_bus] -> slr1_1/1
  slr1_1/1 -> BPAPMWinFOpenedSta/3  "<VINP_CANMsgValidBodyZonePS2_flg>"
  BPAPMWinFOpenedSta/1 -> VINP_BPAPMWinFOpenedSta_pct/1  "VINP_BPAPMWinFOpenedSta_pct"
  BPAPMWinFOpenedSta/2 -> Terminator_1/1
  [BHAL_outputs] -> slr_VHAL_BPAPMWinROpenedSta_pct/1
  slr_VHAL_BPAPMWinROpenedSta_pct/1 -> BPAPMWinROpenedSta/1  "<VHAL_BPAPMWinROpenedSta_pct>"
  True_VHAL_BPAPMWinROpenedSta_pct/1 -> BPAPMWinROpenedSta/2
  [inp_CanValid_bus] -> slr1_2/1
  slr1_2/1 -> BPAPMWinROpenedSta/3  "<VINP_CANMsgValidBodyZonePS2_flg>"
  BPAPMWinROpenedSta/1 -> VINP_BPAPMWinROpenedSta_pct/1  "VINP_BPAPMWinROpenedSta_pct"
  BPAPMWinROpenedSta/2 -> Terminator_2/1
  [BHAL_outputs] -> slr_VHAL_BPDoorFHandleCloseSta_flg/1
  slr_VHAL_BPDoorFHandleCloseSta_flg/1 -> BPDoorFHandleCloseSta/1  "<VHAL_BPDoorFHandleCloseSta_flg>"
  True_VHAL_BPDoorFHandleCloseSta_flg/1 -> BPDoorFHandleCloseSta/2
  [inp_CanValid_bus] -> slr1_3/1
  slr1_3/1 -> BPDoorFHandleCloseSta/3  "<VINP_CANMsgValidBodyZonePS2_flg>"
  BPDoorFHandleCloseSta/1 -> VINP_BPDoorFHandleCloseSta_flg/1  "VINP_BPDoorFHandleCloseSta_flg"
  BPDoorFHandleCloseSta/2 -> Terminator_3/1
  [BHAL_outputs] -> slr_VHAL_BPDoorRHandleCloseSta_flg/1
  slr_VHAL_BPDoorRHandleCloseSta_flg/1 -> BPDoorRHandleCloseSta/1  "<VHAL_BPDoorRHandleCloseSta_flg>"
  True_VHAL_BPDoorRHandleCloseSta_flg/1 -> BPDoorRHandleCloseSta/2
  [inp_CanValid_bus] -> slr1_4/1
  slr1_4/1 -> BPDoorRHandleCloseSta/3  "<VINP_CANMsgValidBodyZonePS2_flg>"
  BPDoorRHandleCloseSta/1 -> VINP_BPDoorRHandleCloseSta_flg/1  "VINP_BPDoorRHandleCloseSta_flg"
  BPDoorRHandleCloseSta/2 -> Terminator_4/1
  [BHAL_outputs] -> slr_VHAL_BPSEATLVentSta_enum/1
  slr_VHAL_BPSEATLVentSta_enum/1 -> BPSEATLVentSta/1  "<VHAL_BPSEATLVentSta_enum>"
  True_VHAL_BPSEATLVentSta_enum/1 -> BPSEATLVentSta/2
  [inp_CanValid_bus] -> slr1_5/1
  slr1_5/1 -> BPSEATLVentSta/3  "<VINP_CANMsgValidBodyZonePS2_flg>"
  BPSEATLVentSta/1 -> VINP_BPSEATLVentSta_enum/1  "VINP_BPSEATLVentSta_enum"
  BPSEATLVentSta/2 -> Terminator_5/1
  [BHAL_outputs] -> slr_VHAL_BPSEATMLVentSta_enum/1
  slr_VHAL_BPSEATMLVentSta_enum/1 -> BPSEATMLVentSta/1  "<VHAL_BPSEATMLVentSta_enum>"
  True_VHAL_BPSEATMLVentSta_enum/1 -> BPSEATMLVentSta/2
  [inp_CanValid_bus] -> slr1_6/1
  slr1_6/1 -> BPSEATMLVentSta/3  "<VINP_CANMsgValidBodyZonePS2_flg>"
  BPSEATMLVentSta/1 -> VINP_BPSEATMLVentSta_enum/1  "VINP_BPSEATMLVentSta_enum"
  BPSEATMLVentSta/2 -> Terminator_6/1
  [BHAL_outputs] -> slr_VHAL_BPSEATMRVentSta_enum/1
  slr_VHAL_BPSEATMRVentSta_enum/1 -> BPSEATMRVentSta/1  "<VHAL_BPSEATMRVentSta_enum>"
  True_VHAL_BPSEATMRVentSta_enum/1 -> BPSEATMRVentSta/2
  [inp_CanValid_bus] -> slr1_7/1
  slr1_7/1 -> BPSEATMRVentSta/3  "<VINP_CANMsgValidBodyZonePS2_flg>"
  BPSEATMRVentSta/1 -> VINP_BPSEATMRVentSta_enum/1  "VINP_BPSEATMRVentSta_enum"
  BPSEATMRVentSta/2 -> Terminator_7/1
  [BHAL_outputs] -> slr_VHAL_BPSEATRVentSta_enum/1
  slr_VHAL_BPSEATRVentSta_enum/1 -> BPSEATRVentSta/1  "<VHAL_BPSEATRVentSta_enum>"
  True_VHAL_BPSEATRVentSta_enum/1 -> BPSEATRVentSta/2
  [inp_CanValid_bus] -> slr1_8/1
  slr1_8/1 -> BPSEATRVentSta/3  "<VINP_CANMsgValidBodyZonePS2_flg>"
  BPSEATRVentSta/1 -> VINP_BPSEATRVentSta_enum/1  "VINP_BPSEATRVentSta_enum"
  BPSEATRVentSta/2 -> Terminator_8/1
